simulink model "robot_simulatie"  (R2015b)
settings: Solver=VariableStepAuto  StartTime=0.0  StopTime=10.0  RelTol=1e-3
values from neighbouring files (symbols this model uses):
  state = [qd; q]    [create_structure.m]    (also in generate_dynamics.m; respectConstVel.m = state - [velError; zeros(size(velError))]; runge_kutta.m = respectConstraint(state); simulate_robot.m = 0*ones(stateN,1))
settings Model: Creator=Michiel  LastModifiedBy=Michiel

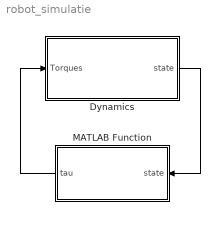
== system robot_simulatie ==
  Dynamics : Subsystem
  MATLAB Function : MATLAB Function  TreatAsAtomicUnit=on
  wires:
  MATLAB Function/1(tau) -> Dynamics/1(Torques)
  Dynamics/1(state) -> MATLAB Function/1(state)

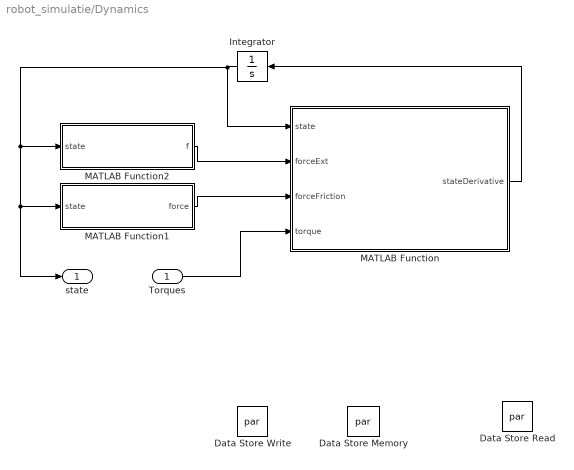
== system robot_simulatie/Dynamics ==
  Torques : Inport
  Data Store Memory : DataStoreMemory  DataStoreName=par  ReadBeforeWriteMsg=warning  WriteAfterWriteMsg=warning  WriteAfterReadMsg=warning
  Data Store Read : DataStoreRead  DataStoreName=par
  Data Store Write : DataStoreWrite  DataStoreName=par
  Integrator : Integrator  InitialCondition=state
  MATLAB Function : MATLAB Function  TreatAsAtomicUnit=on
  MATLAB Function1 : MATLAB Function  TreatAsAtomicUnit=on
  MATLAB Function2 : MATLAB Function  TreatAsAtomicUnit=on
  state : Outport
  wires:
  Integrator/1 -> state/1, MATLAB Function1/1(state), MATLAB Function2/1(state), MATLAB Function/1(state)
  MATLAB Function/1(stateDerivative) -> Integrator/1
  Torques/1 -> MATLAB Function/4(torque)
  MATLAB Function2/1(f) -> MATLAB Function/2(forceExt)
  MATLAB Function1/1(force) -> MATLAB Function/3(forceFriction)

== matlab function robot_simulatie/Dynamics/MATLAB Function1 ==
  data: force output; state input
function force   = computeFriction( state )
%COMPUTEFRICTION Summary of this function goes here
%   Detailed explanation goes here
global par
mu = par.mu;
force = state(length(state)/2+1:end)*mu;
end

== matlab function robot_simulatie/Dynamics/MATLAB Function ==
  data: stateDerivative output; state input; forceExt input; forceFriction input; torque input
function stateDerivative = compute_acceleration(state, forceExt, forceFriction, torque)
    global par
%     t
    u = zeros(length(par.symNames),1);
    if nargin == 3
        u(7:end) = torque;
    else
        u(7:end) = computeTorque(state);
    end
%     state = respectConstVel(state);
    velocity = state(1:length(state)/2);
 
    con = zeros(length(forceExt),length(velocity));
    for i = 1:length(velocity)
        evalString = ['getDoubleJ',par.symNames{i},'(state)'];
        doubleJac = eval(evalString);
        if (~nnz(doubleJac))
            doubleJac = zeros(length(forceExt),length(velocity));
        end
        con(:,i) = doubleJac*velocity;
    end
    J = getJacobian(state);
    
    M = J'*par.M*J;
    
    fw = forceFriction;

    f = u + fw + J'*(par.fz' + forceExt - par.M*con*velocity);
    
    stateDerivative = [M\f; velocity];

== matlab function robot_simulatie/Dynamics/MATLAB Function2 ==
  data: f output; state input
function f = computeContacts(state)

global par

velocity = state(1:length(state)/2);
pContacts = getContactPosition(state);
vContacts = getContactJacobian(state)*velocity;

hLft.i = 1:3;
hRght.i = 7:9;
tLft.i = 4:6;
tRght.i = 10:12;

hLft.p = pContacts(hLft.i);
hRght.p = pContacts(hRght.i);
tLft.p = pContacts(tLft.i);
tRght.p = pContacts(tRght.i);

hLft.v = vContacts(hLft.i);
hRght.v = vContacts(hRght.i);
tLft.v = vContacts(tLft.i);
tRght.v = vContacts(tRght.i);

hLft.f = computeContactForce(hLft.p,hLft.v);
hRght.f = computeContactForce(hRght.p,hRght.v);
tLft.f = computeContactForce(tLft.p,tLft.v);
tRght.f = computeContactForce(tRght.p,tRght.v);

Lft.tau = cross(par.com(:,4),hLft.f) + cross(par.com(:,4)-par.joint(:,4),tLft.f);
Rght.tau = cross(par.com(:,7),hRght.f) + cross(par.com(:,7)-par.joint(:,7),tRght.f);
Lft.F = hLft.f + tLft.f;
Rght.F = hRght.f + tRght.f;

f = zeros(length(par.fz),1);
f(19:24) = [Lft.F; 0*Lft.tau];
f(37:42) = [Rght.F; 0*Rght.tau];

== matlab function robot_simulatie/MATLAB Function ==
  data: state input; tau output
function tau = computeTorque(state)
global par

stateDesired = zeros(length(state),1);

stateDiff = stateDesired - state;
tau = zeros(length(par.symNamesu),1);
if (~isempty(par.Klqr))
    tau(par.linTI) = par.Klqr*stateDiff([par.linSI, length(par.symNames) + par.linSI]);
end
